simulink model "magball_validate_linear"  (Simulink 7.6)
settings: Solver=ode45  StartTime=0.0  StopTime=4  RelTol=1e-3
PreLoadFcn:
  | load magball_validate
libraries: cstblocks x1
settings Model: Creator=The MathWorks Inc.
settings SolverCC: InsertRTBMode=Auto
settings DataIOCC: InitialState=x_struct  LoadInitialState=on
settings OptimizationCC: InitFltsAndDblsToZero=on
settings DebuggingCC: SolverPrmCheckMsg=none  StrictBusMsg=Warning

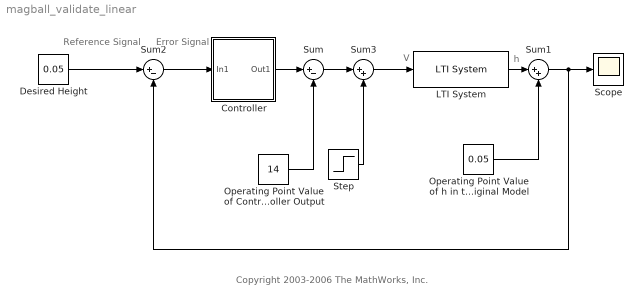
== system magball_validate_linear ==
  note: Error
      | Signal
  note: Reference
      | Signal
  note: V
  note: Copyright 2003-2006 The MathWorks, Inc.
  note: h
  Controller : Subsystem
      settings: RTWMemSecFuncInitTerm=Default  RTWMemSecFuncExecute=Default  RTWMemSecDataConstants=Default  RTWMemSecDataInternal=Default  RTWMemSecDataParameters=Default
  Desired Height : Constant  Value=0.05
  LTI System : cstblocks/LTI System  SystemSampleTime=-1  sys=Model_sys  IC=[]
  Operating Point Value of Controller Output : Constant  Value=14
  Operating Point Value of h in the Original Model : Constant  Value=0.05
  Scope : Scope
      settings: YMin=0.049  YMax=0.0502
  Step : Step  After=2  SampleTime=0
  Sum : Sum  Inputs=|+-
  Sum1 : Sum  Inputs=|++
  Sum2 : Sum  Inputs=|+-
  Sum3 : Sum  Inputs=|++
  wires:
  Sum2/1 -> Controller/1(In1)
  Desired Height/1 -> Sum2/1
  Operating Point Value of Controller Output/1 -> Sum/2
  Operating Point Value of h in the Original Model/1 -> Sum1/2
  Step/1 -> Sum3/2
  Controller/1(Out1) -> Sum/1
  Sum/1 -> Sum3/1
  Sum3/1 -> LTI System/1
  LTI System/1 -> Sum1/1
  Sum1/1 -> Sum2/2, Scope/1

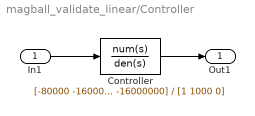
== system magball_validate_linear/Controller ==
  In1 : Inport
  Controller : TransferFcn  Numerator=[-80000 -1600000 -16000000]  Denominator=[1 1000 0]
  Out1 : Outport
  wires:
  In1/1 -> Controller/1
  Controller/1 -> Out1/1
